simulink model "Equivalent_BB_Model"  (R2017a)
settings: Solver=VariableStepDiscrete  StartTime=0.0  StopTime=inf  FixedStep=1/(PSF_SampPerSym*Rsymbol*2)  RelTol=1e-3  EnableMultiTasking=on
PreLoadFcn:
  | %Rates
  | BitRate=(250)*1e3;
  | ChipRate=2e6;
  | SymRate=ChipRate/2;
  | RX_ChipDelay=6;
  | 
  | %Pulse shaping filter
  | OS=32;
  | 
  | Pin=-40;
  | 
  | NF_LNA=4;
  | Gain_LNA=20;
  | 
  | NF_MIX=9;
  | Gain_MIX=-5;
  | 
  | NF_VGA=12;
  | Gain_VGA=44-15;
  | 
  | PLL_NOISE=[-80 -80 -80 -80 -85 -95];
  | PLL_FREQ=[0.01 0.1 1 2 3 7]*1e6;
  | 
  | FLICKER_KERN=2^11;
  | FLICKER_CORNER=10e3;
  | FLICKER_PSD_FLOOR=-124;
  | 
  | fc_RF=2450e6;
InitFcn:
  | x=linspace(0,1,OS);
  | weights=sin(pi*x);
undefined symbols (not defined in the file or in its folder): dBc, dfilt, Hz, read, rfdata
libraries: simulink x3, dspmlti4 x2, dspmathops x2, commdigbbndpm3 x2, dspstat3 x2, commrflib2 x2, rfports1 x2, rfamplifiers1 x2, dspobslib x2, commrandsrc2 x1, commseqgen2 x1, commfilt2 x1
settings Model: Creator=The MathWorks Inc.  LastModifiedBy=gzucchel
settings DataIOCC: LimitDataPoints=on  SaveFormat=Array  SignalLoggingSaveFormat=ModelDataLogs  SaveOutput=off  SignalLogging=off  DSMLogging=off  SaveTime=off
settings OptimizationCC: ExpressionDepthLimit=2147483647  LifeSpan=inf
settings DebuggingCC: UnderspecifiedInitializationDetection=Classic  MergeDetectMultiDrivingBlocksExec=none  SolverPrmCheckMsg=warning  FcnCallInpInsideContextMsg=warning  StateNameClashWarn=warning  SFUnexpectedBacktrackingDiag=warning  SFNoUnconditionalDefaultTransitionDiag=warning  SFExecutionAtInitializationDiag=none
settings HardwareCC: ProdBitPerPointer=32  ProdBitPerSizeT=32  ProdBitPerPtrDiffT=32  ProdLargestAtomicFloat=None  ProdIntDivRoundTo=Undefined  ProdEndianess=Unspecified  ProdWordSize=32  ProdHWDeviceType=32-bit Generic
settings ModelReferenceCC: PropagateSignalLabelsOutOfModel=off
settings GRTTargetCC: TargetLangStandard=C89/C90 (ANSI)  GeneratePreprocessorConditionals=Disable all  CombineOutputUpdateFcns=off  GRTInterface=on
settings ConfigComp: CovMetricSettings=dw  CovHtmlReporting=on  CovSaveCumulativeToWorkspaceVar=on  CovSaveSingleToWorkspaceVar=on  CovExternalEMLEnable=off  CovSFcnEnable=off
settings SimscapeCC: SimscapeNormalizeSystem=off  SimscapeNominalValues="[{\"value\":\"10\",\"unit\":\"V\"},{\"value\":\"1\",\"unit\":\"A\"},{\"value\":\"10\",\"unit\":\"N*m\"},{\"value\":\"10\",\"unit\":\"bar\"},{\"value\":\"100\",\"unit\":\"kJ/kg\"},{\"value\":\"1\",\"unit\":\"kW\"},{\"value\":\"300\",\"unit\":\"K\"},{\"value\":\"100\",\"unit\":\"cm^3/s\"},{\"value\":\"1\",\"unit\":\"kN\"},{\"value\":\"1\",\"unit\":\"g/cm^3\"},{\"value\":\"1\",\"unit\":\"l\"},{\"value\":\"1\",\"unit\":\"cm^2\"},{\"value\":\"60\",\"unit\":\"Hz\"}]"
settings ConfigurationSet: Description=SimMechanics 2G

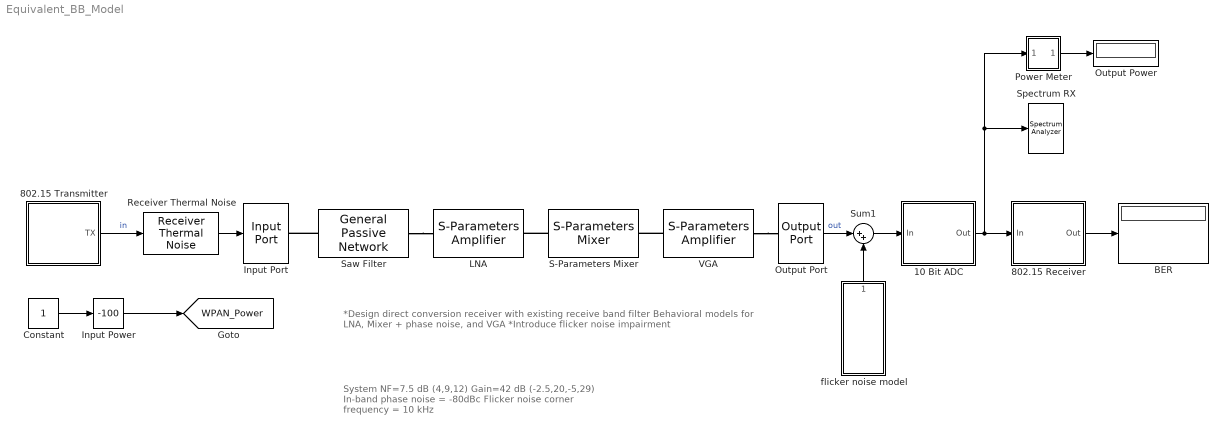
== system Equivalent_BB_Model ==
  note: *Design direct conversion receiver with existing receive band filter
      | Behavioral models for LNA, Mixer + phase noise, and VGA
      | *Introduce flicker noise impairment
  note: System NF=7.5 dB (4,9,12)
      | Gain=42 dB (-2.5,20,-5,29)
      | In-band phase noise = -80dBc
      | Flicker noise corner frequency = 10 kHz
  10 Bit ADC : Subsystem  mask{FS_P_dBm=0, Rnorm=1, N=10, Sample_Rate=0.0}
      mask prompts: FS_P_dBm "Full Scale Power"; Rnorm "Normalization Resistance"; Sample_Rate "Sample Rate (-1 for inherited)"
      mask init:
      | %LSB=FS_V/(2^(N-1));
      | %MAX=FS_V-LSB;
      | %MIN=-FS_V+LSB;
      | LSB=sqrt(2*Rnorm)*sqrt(1e-3)*sqrt(10^(FS_P_dBm/10))/(2^(N-1));
      | MAXp=sqrt(2*Rnorm)*sqrt(1e-3)*sqrt(10^(FS_P_dBm/10))-LSB;
      | MINp=-sqrt(2*Rnorm)*sqrt(1e-3)*sqrt(10^(FS_P_dBm/10))+LSB;
  802.15 Transmitter : Subsystem
  802.15 Receiver : Subsystem
  BER : Display
  Constant : Constant
  Input Port : rfports1/Input Port  Description=source block  TreatSimulinkInputSignalAs=Incident power wave  MaxLength=256  FracBW=0.2  ModelDelay=0  Fc=2.45e9  Ts=1/ChipRate/OS*2  Zs=50  RFhasDSP=Columns as channels (frame based)  NoiseFlag=on  seed=1528  GoToTag=ACCDKBHHIWZHZJZFCRNZWMC
      settings: SourceProductName=RF Toolbox  SourceProductBaseCode=RF
  Input Power : simulink/Math Operations/Slider Gain  gain=-100  low=-120  high=-30
  LNA : rfamplifiers1/S-Parameters Amplifier  LConnTagsString=__newl0  RConnTagsString=__newr0  NetParamData=[0,0;10^(Gain_LNA/20),0]  NetParamFreq=2.45e9  Z0=50  InterpMethod=Linear  IP3Type=OIP3  IIP3=inf  OIP3=inf  P1dB=inf  PSat=inf  GCSat=3  NonlinearDataFreq=2.0e9  NoiseDefinedBy=Noise figure  NF=NF_LNA  FMIN=0  GammaOpt=1+0i  RN=1  NFactor=1  NTemp=0  NoiseDataFreq=2.45e9  PlotFreq=Derived from Input Port parameters  SourceFreq=Same as the s-parameters frequency  Freq=[1.9e9:1.0e8:2.2e9]  SourcePin=Extracted from data source  Pin=0  AllPlotType=X-Y plane  AppliedNetworkData=S11  AppliedComplexFormat=Magnitude (decibels)  AppliedNetworkData2=""  AppliedComplexFormat2=""  AppliedXParameter=Freq  AppliedXFormat=Hz  YOption=Linear  XOption=Linear  PlotZ0=50  PlotFreqNoSim=User-specified  DisplayData=off  NetworkData=S11  SmithData=S11  PolarData=S11  ComplexFormat=Magnitude (decibels)  DBFormat=Magnitude (decibels)  NoneFormat=None
      settings: SourceProductName=RF Toolbox  SourceProductBaseCode=RF
  Output Port : rfports1/Output Port  Zl=50  Flag=0  num_Models=0  GoToTag=ACCDKBHHIWZHZJZFCRNZWMC  PlotFreq=User-specified  SourceFreq=Derived from Input Port parameters  Freq=1e9:1e8:3e9  AllPlotType=X-Y plane  AppliedNetworkData=S11  AppliedComplexFormat=Magnitude (decibels)  AppliedNetworkData2=""  AppliedComplexFormat2=""  AppliedXParameter=Freq  AppliedXFormat=Auto  YOption=Linear  XOption=Linear  PlotZ0=50  DisplayData=off  NoBudgetPlot=Composite data  NetworkData=S11  SmithData=S11  PolarData=S11  ComplexFormat=Magnitude (decibels)  DBFormat=Magnitude (decibels)  DBMFormat=dBm  NoneFormat=None
      settings: SourceProductName=RF Toolbox  SourceProductBaseCode=RF
  Output Power : Display
  Power Meter : Subsystem  mask{R=1, PB=off, buffer_sz=32*32}
      mask prompts: R "Resistance"; PB "Passband Power (Divide by 2)"; buffer_sz "Buffer Size"
  Receiver Thermal Noise : commrflib2/Receiver Thermal Noise  method=Noise temperature  ntemp=290  nfigure=3.01  nfactor=2  add290KAntennaNoise=off  seed=67987
      settings: SourceProductName=Communications System Toolbox  SourceProductBaseCode=CM
  S-Parameters Mixer : rfmixers1/S-Parameters Mixer  LConnTagsString=__newl0  RConnTagsString=__newr0  NetParamData=[0,0;10^(Gain_MIX/20),0]  NetParamFreq=2.45e9  Z0=50  InterpMethod=Linear  MixerType=Downconverter  FLO=2.4e9 %Artificial LO  IP3Type=OIP3  IIP3=inf  OIP3=inf  P1dB=inf  PSat=inf  GCSat=3  NonlinearDataFreq=2.0e9  NoiseDefinedBy=Noise figure  NF=NF_MIX  FMIN=0  GammaOpt=1+0i  RN=1  NFactor=1  NTemp=0  NoiseDataFreq=2.45e9  FreqOffset=PLL_FREQ  PhaseNoiseLevel=PLL_NOISE  PlotFreq=Same as the Frequency parameter  SourceFreq=Same as the s-parameters frequency  Freq=[1e9:1e8:2.9e9]  SourcePin=Extracted from data source  Pin=0  AllPlotType=X-Y plane  AppliedNetworkData=PhaseNoise  AppliedComplexFormat=dBc/Hz  AppliedNetworkData2=""  AppliedComplexFormat2=""  AppliedXParameter=Freq  AppliedXFormat=Hz  YOption=Linear  XOption=Log  PlotZ0=50  PlotFreqNoSim=User-specified  DisplayData=off  NetworkData=S11  SmithData=S11  PolarData=S11  ComplexFormat=Magnitude (decibels)  DBFormat=Magnitude (decibels)  NoneFormat=None  DBcFormat=dBc/Hz
      settings: SourceProductName=RF Toolbox  SourceProductBaseCode=RF
  Saw Filter : rfblackbox1/General Passive Network  LConnTagsString=__newl0  RConnTagsString=__newr0  DataSource=Data file  RFDATA=read(rfdata.data, 'passive.s2p')  File=SAW_Filter_Data.s2p  InterpMethod=Linear  PlotFreq=Extracted from RFDATA object  SourceFreq=Extracted from data source  Freq=[0.3e6:1e7:6e9]  AllPlotType=X-Y plane  AppliedNetworkData=S11  AppliedComplexFormat=Magnitude (decibels)  AppliedNetworkData2=""  AppliedComplexFormat2=""  AppliedXParameter=Freq  AppliedXFormat=Auto  YOption=Linear  XOption=Linear  PlotZ0=50  PlotFreqNoSim=Extracted from RFDATA object  DisplayData=off  NetworkData=S21  SmithData=S11  PolarData=S11  ComplexFormat=Magnitude (decibels)  DBFormat=Magnitude (decibels)  NoneFormat=None
      settings: SourceProductName=RF Toolbox  SourceProductBaseCode=RF
  Spectrum RX : SpectrumAnalyzer
  Sum1 : Sum  Inputs=|++
  VGA : rfamplifiers1/S-Parameters Amplifier  LConnTagsString=__newl0  RConnTagsString=__newr0  NetParamData=[0,0;10^(Gain_VGA/20),0]  NetParamFreq=2.45e9  Z0=50  InterpMethod=Linear  IP3Type=OIP3  IIP3=inf  OIP3=inf  P1dB=inf  PSat=inf  GCSat=3  NonlinearDataFreq=2.0e9  NoiseDefinedBy=Noise figure  NF=NF_VGA  FMIN=0  GammaOpt=1+0i  RN=1  NFactor=1  NTemp=0  NoiseDataFreq=2.45e9  PlotFreq=Derived from Input Port parameters  SourceFreq=Same as the s-parameters frequency  Freq=[1.9e9:1.0e8:2.2e9]  SourcePin=Extracted from data source  Pin=0  AllPlotType=X-Y plane  AppliedNetworkData=S11  AppliedComplexFormat=Magnitude (decibels)  AppliedNetworkData2=""  AppliedComplexFormat2=""  AppliedXParameter=Freq  AppliedXFormat=Hz  YOption=Linear  XOption=Linear  PlotZ0=50  PlotFreqNoSim=User-specified  DisplayData=off  NetworkData=S11  SmithData=S11  PolarData=S11  ComplexFormat=Magnitude (decibels)  DBFormat=Magnitude (decibels)  NoneFormat=None
      settings: SourceProductName=RF Toolbox  SourceProductBaseCode=RF
  flicker noise model : Subsystem
  tag scope: WPAN_Power=global
  wires:
  Receiver Thermal Noise/1 -> Input Port/1
  802.15 Transmitter/1(TX) -> Receiver Thermal Noise/1  "in"
  Input Power/1 -> [WPAN_Power]
  Constant/1 -> Input Power/1
  Output Port/1 -> Sum1/1  "out"
  flicker noise model/1(BB Signal) -> Sum1/2
  10 Bit ADC/1(Out) -> Power Meter/1(In), Spectrum RX/1, 802.15 Receiver/1(In)
  Power Meter/1(Power) -> Output Power/1
  802.15 Receiver/1(Out) -> BER/1
  Sum1/1 -> 10 Bit ADC/1(In)
  connections:
  Saw Filter/LConn1 -- Input Port/RConn1
  Saw Filter/RConn1 -- LNA/LConn1
  S-Parameters Mixer/LConn1 -- LNA/RConn1
  VGA/LConn1 -- S-Parameters Mixer/RConn1
  VGA/RConn1 -- Output Port/LConn1

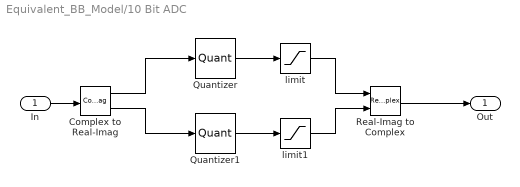
== system Equivalent_BB_Model/10 Bit ADC ==
  In : Inport
  Complex to Real-Imag : ComplexToRealImag
  Quantizer : Quantizer  QuantizationInterval=LSB
  Quantizer1 : Quantizer  QuantizationInterval=LSB
  Real-Imag to Complex : RealImagToComplex
  limit : Saturate  UpperLimit=MAXp  LowerLimit=MINp
  limit1 : Saturate  UpperLimit=MAXp  LowerLimit=MINp
  Out : Outport
  wires:
  Quantizer/1 -> limit/1
  In/1 -> Complex to Real-Imag/1
  Complex to Real-Imag/1 -> Quantizer/1
  Quantizer1/1 -> limit1/1
  Complex to Real-Imag/2 -> Quantizer1/1
  limit/1 -> Real-Imag to Complex/1
  limit1/1 -> Real-Imag to Complex/2
  Real-Imag to Complex/1 -> Out/1

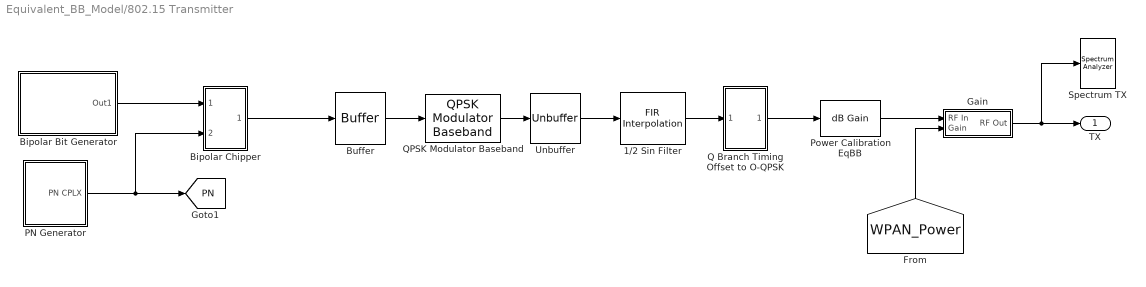
== system Equivalent_BB_Model/802.15 Transmitter ==
  1/2 Sin Filter : dspmlti4/FIR Interpolation  FilterSource=Dialog parameters  h=weights  L=OS  FilterObject=Hm_firinterp  framing=Allow multirate processing  outputBufInitCond=0  roundingMode=Floor  overflowMode=off  firstCoeffDataTypeStr=Inherit: Same word length as input  firstCoeffMin=[]  firstCoeffMax=[]  firstCoeffLastDataTypeStr=Inherit: Same word length as input  outputDataTypeStr=Inherit: Same as accumulator  outputMin=[]  outputMax=[]  outputLastDataTypeStr=Inherit: Same as accumulator
      settings: SourceProductName=DSP System Toolbox
  Bipolar Chipper : Subsystem
  Bipolar Bit Generator : Subsystem
  Buffer : Buffer  N=2
  Gain : Subsystem
  PN Generator : Subsystem
  Power Calibration EqBB : dspmathops/dB Gain  dB=-26.8  intype=Amplitude
      settings: SourceProductName=DSP System Toolbox  SourceProductBaseCode=DS
  Q Branch Timing Offset to O-QPSK : Subsystem
  QPSK Modulator Baseband : commdigbbndpm3/QPSK Modulator Baseband  InType=Bit  Enc=Gray  Ph=pi/4  outDtype=double  outWordLen=16  outUDDataType=sfix(16)  outFracLenMode=Best precision  outFracLen=15  outDataTypeStr=double  outLastDataTypeStr=double
  Spectrum TX : SpectrumAnalyzer
  Unbuffer : Unbuffer
  TX : Outport
  tag scope: PN=global
  wires:
  QPSK Modulator Baseband/1 -> Unbuffer/1
  1/2 Sin Filter/1 -> Q Branch Timing Offset to O-QPSK/1(In1)
  PN Generator/1(PN CPLX) -> Bipolar Chipper/2(In2), [PN]
  Bipolar Bit Generator/1(Out1) -> Bipolar Chipper/1(In1)
  Bipolar Chipper/1(Out1) -> Buffer/1
  Buffer/1 -> QPSK Modulator Baseband/1
  Unbuffer/1 -> 1/2 Sin Filter/1
  [WPAN_Power] -> Gain/2(Gain)
  Gain/1(RF Out) -> TX/1, Spectrum TX/1
  Q Branch Timing Offset to O-QPSK/1(Out1) -> Power Calibration EqBB/1
  Power Calibration EqBB/1 -> Gain/1(RF In)

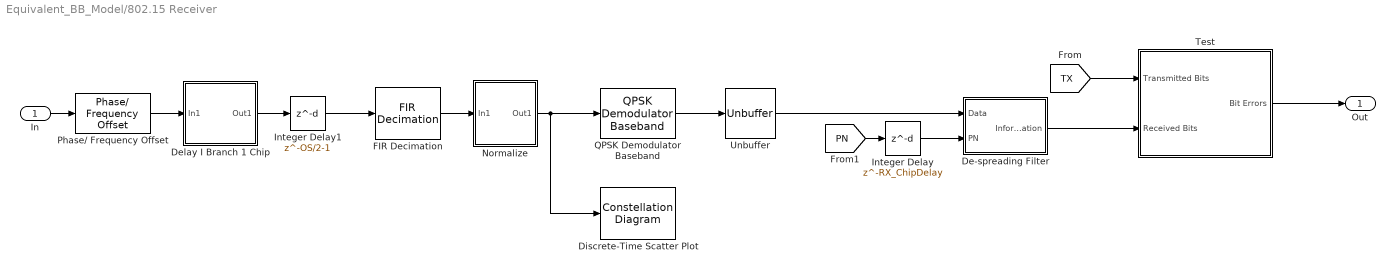
== system Equivalent_BB_Model/802.15 Receiver ==
  In : Inport
  De-spreading Filter : Subsystem
  Delay I Branch 1 Chip : Subsystem
  Discrete-Time Scatter Plot : ConstellationDiagram  Tag=ScatterPlot
  FIR Decimation : dspmlti4/FIR Decimation  FilterSource=Dialog parameters  h=fliplr(conj(weights))  D=OS  filtStruct=Direct form  FilterObject=Hm_firdecim  InputProcessing=Columns as channels (frame based)  framing=Allow multirate processing  inputOffset=0  outputBufInitCond=0  roundingMode=Floor  overflowMode=off  firstCoeffDataTypeStr=Inherit: Same word length as input  firstCoeffMin=[]  firstCoeffMax=[]  firstCoeffLastDataTypeStr=Inherit: Same word length as input  outputDataTypeStr=Inherit: Same as accumulator  outputMin=[]  outputMax=[]  outputLastDataTypeStr=Inherit: Same as accumulator
  Integer Delay : Delay  DelayLength=RX_ChipDelay
  Integer Delay1 : Delay  DelayLength=OS/2-1
  Normalize : Subsystem
  Phase/ Frequency Offset : commrflib2/Phase// Frequency Offset  phaseOffset=57  freqPort=off  freqOffset=0
      settings: SourceProductName=Communications System Toolbox
  QPSK Demodulator Baseband : commdigbbndpm3/QPSK Demodulator Baseband  OutType=Bit  DecType=Hard decision  VarSource=Dialog  Variance=1  Dec=Gray  Ph=pi/4  outDtype1=Inherit via internal rule  outDtype2=Inherit via internal rule  derotateFactorWordLen=16  derotateFactorDataTypeStr=Inherit: Same word length as input  derotateFactorLastDataTypeStr=Inherit: Same word length as input
  Test : Subsystem
  Unbuffer : Unbuffer
  Out : Outport
  wires:
  De-spreading Filter/1(Information) -> Test/2(Received Bits)
  Integer Delay/1 -> De-spreading Filter/2(PN)
  [PN] -> Integer Delay/1
  Unbuffer/1 -> De-spreading Filter/1(Data)
  Normalize/1(Out1) -> QPSK Demodulator Baseband/1, Discrete-Time Scatter Plot/1
  Integer Delay1/1 -> FIR Decimation/1
  FIR Decimation/1 -> Normalize/1(In1)
  QPSK Demodulator Baseband/1 -> Unbuffer/1
  In/1 -> Phase/ Frequency Offset/1
  Delay I Branch 1 Chip/1(Out1) -> Integer Delay1/1
  Test/1(Bit Errors) -> Out/1
  [TX] -> Test/1(Transmitted Bits)
  Phase/ Frequency Offset/1 -> Delay I Branch 1 Chip/1(In1)

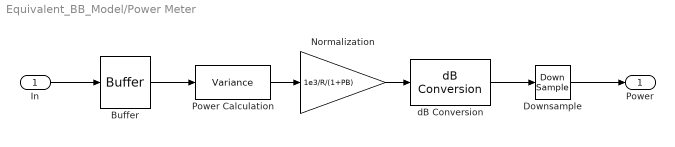
== system Equivalent_BB_Model/Power Meter ==
  In : Inport
  Buffer : Buffer  N=buffer_sz
  Downsample : DownSample  N=10  RateOptions=Allow multirate processing
  Normalization : Gain  Gain=1e3/R/(1+PB)
  Power Calculation : dspstat3/Variance  run=off  reset_popup=None  InputProcessing=Columns as channels (frame based)  directionMode=Each column  dimension=1  roiEnable=off  roiType=Rectangles  roiPortion=Entire ROI  roiOutput=Individual statistics for each ROI  roiFlag=off  roundingMode=Floor  overflowMode=off
      settings: SourceProductName=DSP System Toolbox
  dB Conversion : dspmathops/dB Conversion  dBtype=dB  intype=Power  R=1  fuzz=on
      settings: SourceProductName=DSP System Toolbox
  Power : Outport
  wires:
  dB Conversion/1 -> Downsample/1
  Buffer/1 -> Power Calculation/1
  In/1 -> Buffer/1
  Normalization/1 -> dB Conversion/1
  Power Calculation/1 -> Normalization/1
  Downsample/1 -> Power/1

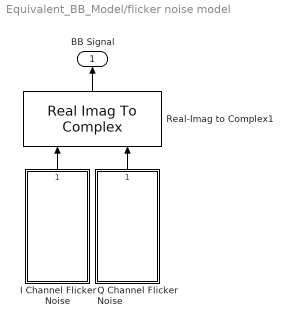
== system Equivalent_BB_Model/flicker noise model ==
  I Channel Flicker Noise : Subsystem  mask{Npts=FLICKER_KERN, Fs=SymRate*OS, fcorner=FLICKER_CORNER, Pcorner_dBm=FLICKER_PSD_FLOOR, R=1, seed=12345}
      mask prompts: Npts "Filter Kernel Size"; Fs "Sampling Frequency (Hz)"; fcorner "Flicker Noise Corner Frequency (Hz)"; Pcorner_dBm "Single Sided System Noise Floor (dBm/Hz)"; R "Reference Impedance"; seed "Random Seed"
      mask init:
      | noise_filt=pinkNoise(Npts, Fs, fcorner, Pcorner_dBm,R);
  Q Channel Flicker Noise : Subsystem  mask{Npts=FLICKER_KERN, Fs=SymRate*OS, fcorner=FLICKER_CORNER, Pcorner_dBm=FLICKER_PSD_FLOOR, R=1, seed=67543}
      mask prompts: Npts "Filter Kernel Size"; Fs "Sampling Frequency (Hz)"; fcorner "Flicker Noise Corner Frequency (Hz)"; Pcorner_dBm "Single Sided System Noise Floor (dBm/Hz)"; R "Reference Impedance"; seed "Random Seed"
      mask init:
      | noise_filt=pinkNoise(Npts, Fs, fcorner, Pcorner_dBm,R);
  Real-Imag to Complex1 : RealImagToComplex
  BB Signal : Outport
  wires:
  I Channel Flicker Noise/1(Baseband Noise) -> Real-Imag to Complex1/1
  Q Channel Flicker Noise/1(Baseband Noise) -> Real-Imag to Complex1/2
  Real-Imag to Complex1/1 -> BB Signal/1

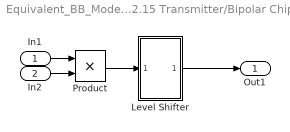
== system Equivalent_BB_Model/802.15 Transmitter/Bipolar Chipper ==
  In1 : Inport
  In2 : Inport  Port=2
  Level Shifter : Subsystem
  Product : Product  RndMeth=Zero
  Out1 : Outport
  wires:
  In2/1 -> Product/2
  Level Shifter/1(Out1) -> Out1/1
  In1/1 -> Product/1
  Product/1 -> Level Shifter/1(In1)

== system Equivalent_BB_Model/802.15 Transmitter/Bipolar Bit Generator ==
  Bernoulli Binary Generator : commrandsrc2/Bernoulli Binary Generator  P=0.5  seed=61  Ts=1/BitRate  frameBased=off  sampPerFrame=1  orient=off  outDataType=double
  Level Shifter : Subsystem
  Out1 : Outport
  tag scope: TX=global
  wires:
  Level Shifter/1(Out1) -> Out1/1
  Bernoulli Binary Generator/1 -> [TX], Level Shifter/1(In1)

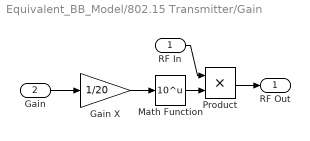
== system Equivalent_BB_Model/802.15 Transmitter/Gain ==
  RF In : Inport
  Gain : Inport  Port=2
  Gain X : Gain  Gain=1/20
  Math Function : Math  Operator=10^u  SaturateOnIntegerOverflow=on
  Product : Product  RndMeth=Zero
  RF Out : Outport
  wires:
  Gain/1 -> Gain X/1
  Product/1 -> RF Out/1
  RF In/1 -> Product/1
  Math Function/1 -> Product/2
  Gain X/1 -> Math Function/1

== system Equivalent_BB_Model/802.15 Transmitter/PN Generator ==
  Level Shifter : Subsystem
  Scrambling code : commseqgen2/PN Sequence Generator  poly=[0 -7 -10]  ini_sta=[1 0 0 0 0 0 0 0 0 0]  outBitMaskSource=Dialog parameter  shift=0  outVarSiz=off  maxOutSizeMode=Dialog parameter  maxOutSize=[10 1]  Ts=1/ChipRate  frameBased=off  sampPerFrame=1  reset=off  bitPackedOutputs=off  outDataType=double  numPackedBits=8  bitPackDataSigned=off  bitPackedOutDType=double
  PN CPLX : Outport
  wires:
  Level Shifter/1(Out1) -> PN CPLX/1
  Scrambling code/1 -> Level Shifter/1(In1)

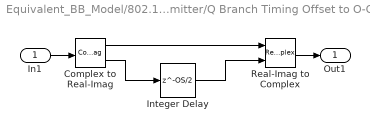
== system Equivalent_BB_Model/802.15 Transmitter/Q Branch Timing Offset to O-QPSK ==
  In1 : Inport
  Complex to Real-Imag : ComplexToRealImag
  Integer Delay : Delay  DelayLength=OS/2
  Real-Imag to Complex : RealImagToComplex
  Out1 : Outport
  wires:
  Real-Imag to Complex/1 -> Out1/1
  In1/1 -> Complex to Real-Imag/1
  Complex to Real-Imag/1 -> Real-Imag to Complex/1
  Integer Delay/1 -> Real-Imag to Complex/2
  Complex to Real-Imag/2 -> Integer Delay/1

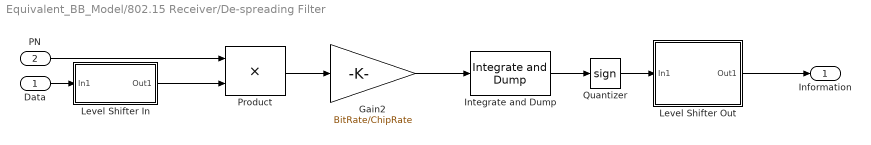
== system Equivalent_BB_Model/802.15 Receiver/De-spreading Filter ==
  Data : Inport
  PN : Inport  Port=2
  Gain2 : Gain  Gain=BitRate/ChipRate  SaturateOnIntegerOverflow=on  OutDataTypeStr=Inherit: Same as input  ParamDataTypeStr=Inherit: Same as input
  Integrate and Dump : commfilt2/Integrate and Dump  obssamples=ChipRate/BitRate  offsetsamples=RX_ChipDelay  nodump=off  roundingMode=Floor  overflowMode=off  outputDataTypeStr=Inherit: Same as accumulator  outputLastDataTypeStr=Inherit: Same as accumulator
      settings: SourceProductName=Communications System Toolbox
  Level Shifter In : Subsystem
  Level Shifter Out : Subsystem
  Product : Product  RndMeth=Zero
  Quantizer : Signum
  Information : Outport
  wires:
  Quantizer/1 -> Level Shifter Out/1(In1)
  PN/1 -> Product/1
  Integrate and Dump/1 -> Quantizer/1
  Level Shifter In/1(Out1) -> Product/2
  Product/1 -> Gain2/1
  Gain2/1 -> Integrate and Dump/1
  Level Shifter Out/1(Out1) -> Information/1
  Data/1 -> Level Shifter In/1(In1)

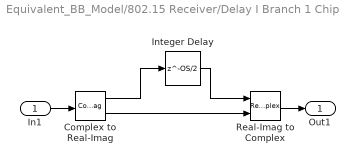
== system Equivalent_BB_Model/802.15 Receiver/Delay I Branch 1 Chip ==
  In1 : Inport
  Complex to Real-Imag : ComplexToRealImag
  Integer Delay : Delay  DelayLength=OS/2
  Real-Imag to Complex : RealImagToComplex
  Out1 : Outport
  wires:
  Real-Imag to Complex/1 -> Out1/1
  In1/1 -> Complex to Real-Imag/1
  Complex to Real-Imag/2 -> Real-Imag to Complex/2
  Integer Delay/1 -> Real-Imag to Complex/1
  Complex to Real-Imag/1 -> Integer Delay/1

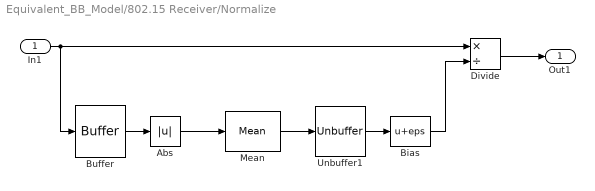
== system Equivalent_BB_Model/802.15 Receiver/Normalize ==
  In1 : Inport
  Abs : Abs
  Bias : Bias  Bias=eps
  Buffer : Buffer
  Divide : Product  Inputs=*/
  Mean : dspstat3/Mean  run=off  reset_popup=None  InputProcessing=Columns as channels (frame based)  directionMode=Each column  dimension=1  roiEnable=off  roiType=Rectangles  roiPortion=Entire ROI  roiOutput=Individual statistics for each ROI  roiFlag=off  outputDataTypeStr=Inherit: Same as accumulator  outputLastDataTypeStr=Inherit: Same as accumulator  outputMin=[]  outputMax=[]  roundingMode=Floor  overflowMode=off
  Unbuffer1 : Unbuffer
  Out1 : Outport
  wires:
  Bias/1 -> Divide/2
  Unbuffer1/1 -> Bias/1
  Divide/1 -> Out1/1
  In1/1 -> Divide/1, Buffer/1
  Mean/1 -> Unbuffer1/1
  Abs/1 -> Mean/1
  Buffer/1 -> Abs/1

== system Equivalent_BB_Model/802.15 Receiver/Test ==
  Transmitted Bits : Inport
  Received Bits : Inport  Port=2
  Error Rate Calculation : commsink2/Error Rate Calculation  N=2  st_delay=2  cp_mode=Entire frame  subframe=[]  PMode=Port  WsName=ErrorVec  RsMode2=off  stop=off  numErr=inf  maxBits=20000
  Bit Errors : Outport
  wires:
  Received Bits/1 -> Error Rate Calculation/2
  Error Rate Calculation/1 -> Bit Errors/1
  Transmitted Bits/1 -> Error Rate Calculation/1

== system Equivalent_BB_Model/flicker noise model/I Channel Flicker Noise ==
  Band-Limited White Noise : simulink/Sources/Band-Limited White Noise  Cov=1  Ts=1/Fs  seed=seed
  Digital Filter : dspobslib/Digital Filter  TypePopup=FIR (all zeros)  IIRFiltStruct=Direct form II  AllPoleFiltStruct=Direct form  FIRFiltStruct=Direct form  CoeffSource=Specify via dialog  NumCoeffs=noise_filt  DenCoeffs=a  BiQuadCoeffs=[1 0.3 0.4 1 0.1 0.2]  LatticeCoeffs=[0.2 0.4]  denIgnore=on  FiltPerSampPopup=One filter per frame  IC=0  ICnum=0  ICden=0  roundingMode=Floor  overflowMode=off  ScaleValues=1  scaleValueFracLength=14  stageInFracLength=15  stageOutFracLength=15  FilterSource=Specify via dialog  dfiltObjectName=dfilt.dffir([1 2 1])
      settings: SourceProductName=DSP System Toolbox  SourceProductBaseCode=DS
  Baseband Noise : Outport
  wires:
  Band-Limited White Noise/1 -> Digital Filter/1
  Digital Filter/1 -> Baseband Noise/1

== system Equivalent_BB_Model/flicker noise model/Q Channel Flicker Noise ==
  Band-Limited White Noise : simulink/Sources/Band-Limited White Noise  Cov=1  Ts=1/Fs  seed=seed
  Digital Filter : dspobslib/Digital Filter  TypePopup=FIR (all zeros)  IIRFiltStruct=Direct form II  AllPoleFiltStruct=Direct form  FIRFiltStruct=Direct form  CoeffSource=Specify via dialog  NumCoeffs=noise_filt  DenCoeffs=a  BiQuadCoeffs=[1 0.3 0.4 1 0.1 0.2]  LatticeCoeffs=[0.2 0.4]  denIgnore=on  FiltPerSampPopup=One filter per frame  IC=0  ICnum=0  ICden=0  roundingMode=Floor  overflowMode=off  ScaleValues=1  scaleValueFracLength=14  stageInFracLength=15  stageOutFracLength=15  FilterSource=Specify via dialog  dfiltObjectName=dfilt.dffir([1 2 1])
      settings: SourceProductName=DSP System Toolbox  SourceProductBaseCode=DS
  Baseband Noise : Outport
  wires:
  Digital Filter/1 -> Baseband Noise/1
  Band-Limited White Noise/1 -> Digital Filter/1

== system Equivalent_BB_Model/802.15 Transmitter/Bipolar Chipper/Level Shifter ==
  In1 : Inport
  Bias : Bias  Bias=1
  Gain : Gain  Gain=0.5
  Out1 : Outport
  wires:
  Gain/1 -> Out1/1
  In1/1 -> Bias/1
  Bias/1 -> Gain/1

== system Equivalent_BB_Model/802.15 Transmitter/Bipolar Bit Generator/Level Shifter ==
  In1 : Inport
  Bias : Bias  Bias=-1
  Gain : Gain  Gain=2
  Out1 : Outport
  wires:
  Bias/1 -> Out1/1
  In1/1 -> Gain/1
  Gain/1 -> Bias/1

== system Equivalent_BB_Model/802.15 Transmitter/PN Generator/Level Shifter ==
  In1 : Inport
  Bias : Bias  Bias=-1
  Gain : Gain  Gain=2
  Out1 : Outport
  wires:
  In1/1 -> Gain/1
  Bias/1 -> Out1/1
  Gain/1 -> Bias/1

== system Equivalent_BB_Model/802.15 Receiver/De-spreading Filter/Level Shifter In ==
  In1 : Inport
  Bias : Bias  Bias=-1
  Gain : Gain  Gain=2
  Out1 : Outport
  wires:
  In1/1 -> Gain/1
  Bias/1 -> Out1/1
  Gain/1 -> Bias/1

== system Equivalent_BB_Model/802.15 Receiver/De-spreading Filter/Level Shifter Out ==
  In1 : Inport
  Bias1 : Bias  Bias=1
  Gain1 : Gain  Gain=0.5
  Out1 : Outport
  wires:
  Gain1/1 -> Out1/1
  In1/1 -> Bias1/1
  Bias1/1 -> Gain1/1
